simulink model "W1P2"  (R2020b)
settings: Solver=VariableStepAuto  StartTime=0.0  StopTime=10.0  RelTol=1e-3
undefined symbols (not defined in the file): b, k1, k2, m1, m2
settings Model: Creator=saadh  LastModifiedBy=saadh

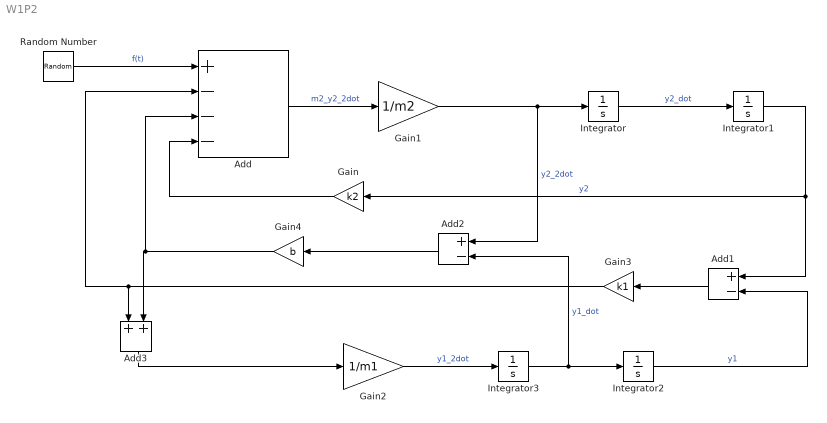
== system W1P2 ==
  Add : Sum  Inputs=+---
  Add1 : Sum  Inputs=+-
  Add2 : Sum  Inputs=+-
  Add3 : Sum
  Gain : Gain  Gain=k2
  Gain1 : Gain  Gain=1/m2
  Gain2 : Gain  Gain=1/m1
  Gain3 : Gain  Gain=k1
  Gain4 : Gain  Gain=b
  Integrator{,1..3} (4 alike) : Integrator
  Random Number : RandomNumber  SampleTime=0.1
  wires:
  Random Number/1 -> Add/1  "f(t)"
  Integrator/1 -> Integrator1/1  "y2_dot"
  Add/1 -> Gain1/1  "m2_y2_2dot"
  Gain1/1 -> Add2/1, Integrator/1  "y2_2dot"
  Integrator1/1 -> Add1/1, Gain/1  "y2"
  Integrator2/1 -> Add1/2  "y1"
  Integrator3/1 -> Add2/2, Integrator2/1  "y1_dot"
  Gain2/1 -> Integrator3/1  "y1_2dot"
  Add1/1 -> Gain3/1
  Gain3/1 -> Add3/1, Add/2
  Gain/1 -> Add/4
  Add2/1 -> Gain4/1
  Gain4/1 -> Add3/2, Add/3
  Add3/1 -> Gain2/1
